simulink model "sсheme"  (R2018b)
settings: Solver=VariableStepAuto  StartTime=0.0  StopTime=20.0  RelTol=1e-3
libraries: dspsrcs4 x2
settings Model: Creator=andrewbelyaev  LastModifiedBy=andrewbelyaev

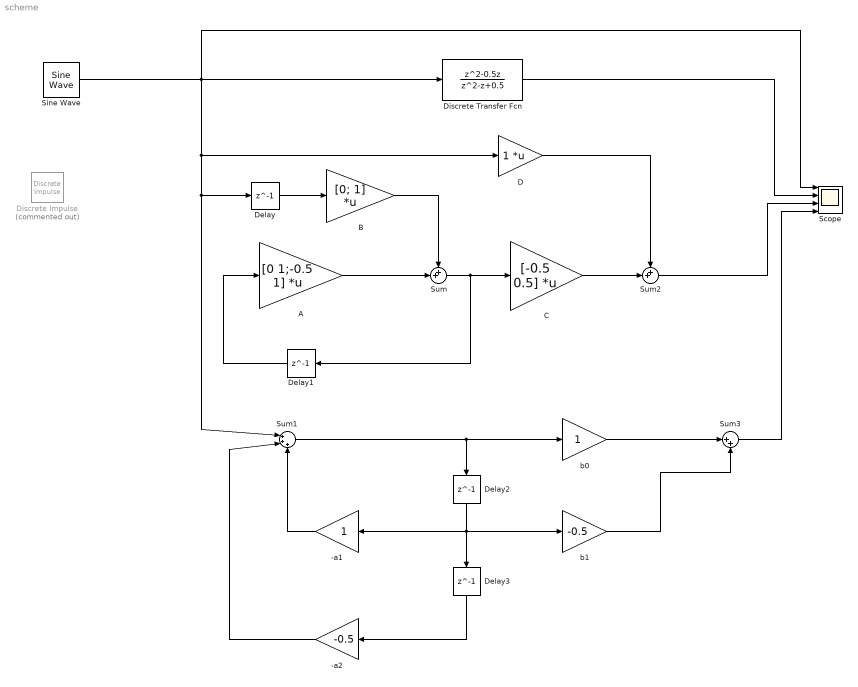
== system sсheme ==
  -a1 : Gain
  -a2 : Gain  Gain=-0.5
  A : Gain  Gain=[0 1;-0.5 1]  Multiplication=Matrix(K*u)
  B : Gain  Gain=[0; 1]  Multiplication=Matrix(K*u)
  C : Gain  Gain=[-0.5 0.5]  Multiplication=Matrix(K*u)
  D : Gain  Multiplication=Matrix(K*u)
  Delay{,1..3} (4 alike) : Delay  DelayLength=1  InitialCondition=0
  Discrete Transfer Fcn : DiscreteTransferFcn  Numerator=[1 -0.5 0]  Denominator=[1 -1 0.5]
  Discrete Impulse : dspsrcs4/Discrete  Impulse  Commented=on  Delay=0  SampleTime=1  FrameSample=1  OutputFrames=off  dataType=double  isSigned=on  wordLen=16  udDataType=sfix(16)  fracBitsMode=Best precision  numFracBits=15  OutDataTypeStr=double  LastOutDataTypeStr=double
  Scope : Scope  NumInputPorts=4
  Sine Wave : dspsrcs4/Sine Wave  Amplitude=1  Frequency=0.2  Phase=pi/2  SampleMode=Discrete  OutComplex=Real  CompMethod=Trigonometric fcn  TableSize=Speed  SampleTime=1/1000  SamplesPerFrame=1  ResetState=Restart at time zero  OutputFrames=off  dataType=double  wordLen=16  udDataType=sfix(16)  fracBitsMode=Best precision  numFracBits=15  OutDataTypeStr=double  LastOutDataTypeStr=double
  Sum : Sum  Inputs=++|
  Sum1 : Sum  Inputs=|+++
  Sum2 : Sum  Inputs=++|
  Sum3 : Sum  Inputs=|++
  b0 : Gain
  b1 : Gain  Gain=-0.5
  wires:
  Discrete Transfer Fcn/1 -> Scope/2
  Delay/1 -> B/1
  B/1 -> Sum/1
  A/1 -> Sum/2
  Delay1/1 -> A/1
  Sum/1 -> Delay1/1, C/1
  C/1 -> Sum2/2
  D/1 -> Sum2/1
  Sum2/1 -> Scope/3
  Delay2/1 -> -a1/1, b1/1, Delay3/1
  Delay3/1 -> -a2/1
  -a2/1 -> Sum1/2
  -a1/1 -> Sum1/3
  Sine Wave/1 -> D/1, Sum1/1, Delay/1, Scope/1, Discrete Transfer Fcn/1
  Sum1/1 -> Delay2/1, b0/1
  b0/1 -> Sum3/1
  b1/1 -> Sum3/2
  Sum3/1 -> Scope/4
